simulink model "gm_wifi_server"  (R2015b)
settings: Solver=VariableStepAuto  StartTime=0.0  StopTime=10.0  RelTol=1e-3
settings Model: Creator=Administrator  LastModifiedBy=Administrator
settings OptimizationCC: BlockReduction=off  ConditionallyExecuteInputs=off
settings DebuggingCC: InheritedTsInSrcMsg=none

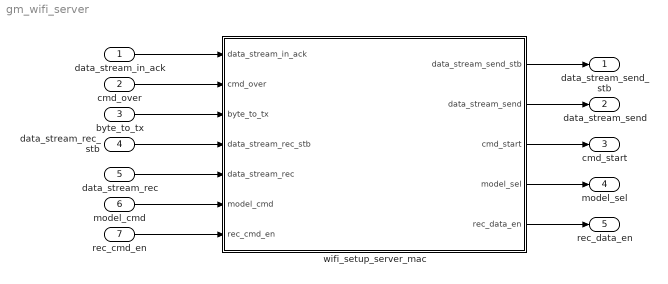
== system gm_wifi_server ==
  data_stream_in_ack : Inport  SampleTime=0
  cmd_over : Inport  Port=2  SampleTime=0
  byte_to_tx : Inport  Port=3  SampleTime=0
  data_stream_rec_stb : Inport  Port=4  SampleTime=0
  data_stream_rec : Inport  Port=5  SampleTime=0
  model_cmd : Inport  Port=6  SampleTime=0
  rec_cmd_en : Inport  Port=7  SampleTime=0
  wifi_setup_server_mac : Subsystem
  data_stream_send_stb : Outport
  data_stream_send : Outport  Port=2
  cmd_start : Outport  Port=3
  model_sel : Outport  Port=4
  rec_data_en : Outport  Port=5
  wires:
  data_stream_in_ack/1 -> wifi_setup_server_mac/1(data_stream_in_ack)
  cmd_over/1 -> wifi_setup_server_mac/2(cmd_over)
  byte_to_tx/1 -> wifi_setup_server_mac/3(byte_to_tx)
  data_stream_rec_stb/1 -> wifi_setup_server_mac/4(data_stream_rec_stb)
  data_stream_rec/1 -> wifi_setup_server_mac/5(data_stream_rec)
  model_cmd/1 -> wifi_setup_server_mac/6(model_cmd)
  rec_cmd_en/1 -> wifi_setup_server_mac/7(rec_cmd_en)
  wifi_setup_server_mac/1(data_stream_send_stb) -> data_stream_send_stb/1
  wifi_setup_server_mac/2(data_stream_send) -> data_stream_send/1
  wifi_setup_server_mac/3(cmd_start) -> cmd_start/1
  wifi_setup_server_mac/4(model_sel) -> model_sel/1
  wifi_setup_server_mac/5(rec_data_en) -> rec_data_en/1

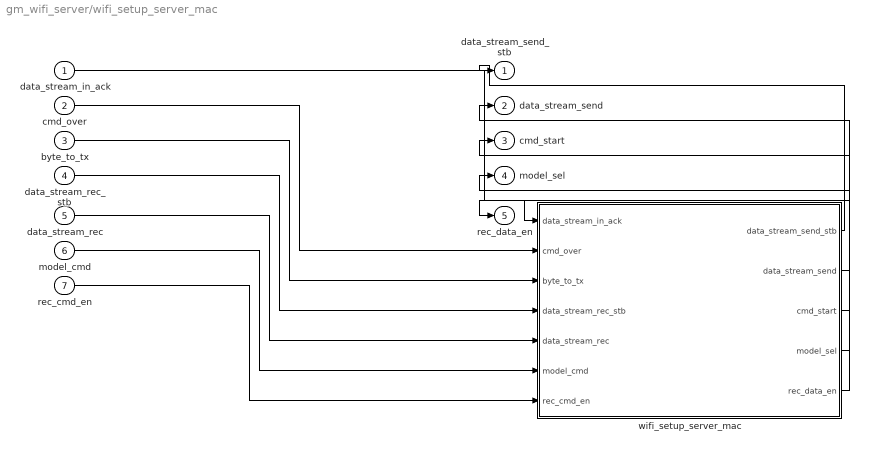
== system gm_wifi_server/wifi_setup_server_mac ==
  data_stream_in_ack : Inport  SampleTime=0
  cmd_over : Inport  Port=2  SampleTime=0
  byte_to_tx : Inport  Port=3  SampleTime=0
  data_stream_rec_stb : Inport  Port=4  SampleTime=0
  data_stream_rec : Inport  Port=5  SampleTime=0
  model_cmd : Inport  Port=6  SampleTime=0
  rec_cmd_en : Inport  Port=7  SampleTime=0
  wifi_setup_server_mac : Stateflow chart  TreatAsAtomicUnit=on
  data_stream_send_stb : Outport
  data_stream_send : Outport  Port=2
  cmd_start : Outport  Port=3
  model_sel : Outport  Port=4
  rec_data_en : Outport  Port=5
  wires:
  data_stream_in_ack/1 -> wifi_setup_server_mac/1(data_stream_in_ack)
  cmd_over/1 -> wifi_setup_server_mac/2(cmd_over)
  byte_to_tx/1 -> wifi_setup_server_mac/3(byte_to_tx)
  data_stream_rec_stb/1 -> wifi_setup_server_mac/4(data_stream_rec_stb)
  data_stream_rec/1 -> wifi_setup_server_mac/5(data_stream_rec)
  model_cmd/1 -> wifi_setup_server_mac/6(model_cmd)
  rec_cmd_en/1 -> wifi_setup_server_mac/7(rec_cmd_en)
  wifi_setup_server_mac/1(data_stream_send_stb) -> data_stream_send_stb/1
  wifi_setup_server_mac/2(data_stream_send) -> data_stream_send/1
  wifi_setup_server_mac/3(cmd_start) -> cmd_start/1
  wifi_setup_server_mac/4(model_sel) -> model_sel/1
  wifi_setup_server_mac/5(rec_data_en) -> rec_data_en/1

== stateflow chart gm_wifi_server/wifi_setup_server_mac/wifi_setup_server_mac ==
  settings: executeAtInitialization=1
  state initial
    entry:
    %outputs
    data_stream_send_stb=0;
    data_stream_send=0;
    cmd_start=0;
    model_sel=0;
    rec_data_en=0;
    %local variables
    cnt_wait=0;
    cnt_halt=0;
  state Tran1_A
    entry:
    data_stream_send_stb=1;
    data_stream_send=65;%A
    cnt_wait=0;
    cnt_halt=0;
  state Tran1_T
    entry:
    data_stream_send_stb=1;
    data_stream_send=84;%T
    cnt_wait=0;
    cnt_halt=0;
  state Tran1_Enter1
    entry:
    data_stream_send_stb=1;
    data_stream_send=10;%/n
    cnt_wait=0;
    cnt_halt=0;
  state Tran1_Enter
    entry:
    data_stream_send_stb=1;
    data_stream_send=13;%/r
    cnt_wait=0;
    cnt_halt=0;
  state send1_finish
    entry:
    data_stream_send_stb=0;
    data_stream_send=0;
    cnt_wait=0;
    cnt_halt=0;
  state wait1_cnt
    cnt_wait=cnt_wait+1;
    cnt_halt=0;
  state send_cmd1
    entry:
    %output
    cmd_start=1;
    data_stream_send_stb=0;
    data_stream_send=byte_to_tx;
    %local
    %cnt_wait=0;
    %cnt_halt=0;
  state send_cmd2
    entry:
    %output
    cmd_start=1;
    data_stream_send_stb=1;
    data_stream_send=byte_to_tx;
  state wait_cmd
    entry:
    cmd_start=1;
    data_stream_send_stb=1;
    data_stream_send=byte_to_tx;
  state device_OK
    entry:
    %output, start from 1
    model_sel=model_sel+1;
    cnt_wait=0;
  state send_cmd_over
    entry:
    cmd_start=0;
    data_stream_send_stb=0;
    data_stream_send=0;
  state Tran2_Enter
    entry:
    data_stream_send_stb=1;
    data_stream_send=13;%/r
  state Tran2_Enter1
    entry:
    data_stream_send_stb=1;
    data_stream_send=10;%/r
  state send2_finish
    entry:
    data_stream_send_stb=0;
    data_stream_send=0;
  state device_config_OK
    entry:
    model_sel=6;
    cnt_halt=0;
  state wait_port
    entry:
    rec_data_en=0;
    cnt_halt=cnt_halt+1;
  state wait_server_rec_S
    entry:
    cnt_halt=cnt_halt+1;
  state wait_server_rec_T
    entry:
    rec_data_en=1;
    %when get T, begin rec data
  state rec_data
    entry:
    cnt_halt=cnt_halt+1;
  state pre_rec_data
  state send_word
    entry:
    cmd_start=1;
    data_stream_send_stb=0;
    data_stream_send=byte_to_tx;
    cnt_halt=0;
  state send_word1
    entry:
    cmd_start=1;
    data_stream_send_stb=1;
    data_stream_send=byte_to_tx;
  state wait_data
    entry:
    cmd_start=1;
    data_stream_send_stb=1;
    data_stream_send=byte_to_tx;
  state begin_send_data
    entry:
    model_sel=7;
    cnt_halt=0;
  state send_data_over
    entry:
    cmd_start=0;
    data_stream_send_stb=0;
    data_stream_send=0;
  state Tran3_Enter
    entry:
    data_stream_send_stb=1;
    data_stream_send=13;%/r
  state Tran3_Enter1
    entry:
    data_stream_send_stb=1;
    data_stream_send=10;%/r
  state send3_finish
    entry:
    data_stream_send_stb=0;
    data_stream_send=0;
  state data_send_over
    entry:
    model_sel=7;
    cnt_halt=0;
  (default) -> initial
  initial -> Tran1_A
  Tran1_A -> (junction 17)
  (junction 17) -> Tran1_T [order 2] : [data_stream_in_ack==1]
  Tran1_T -> (junction 29)
  (junction 29) -> Tran1_Enter [order 1] : [data_stream_in_ack==1]
  Tran1_Enter -> (junction 31)
  (junction 31) -> Tran1_Enter1 [order 1] : [data_stream_in_ack==1]
  (junction 29) -> Tran1_T [order 2] : [data_stream_in_ack==0]
  (junction 31) -> Tran1_Enter [order 2] : [data_stream_in_ack==0]
  (junction 17) -> Tran1_A [order 1] : [data_stream_in_ack==0]
  (junction 42) -> Tran1_Enter1 [order 1] : [data_stream_in_ack==0]
  (junction 49) -> Tran1_A [order 1] : [model_cmd~=1]
  Tran1_Enter1 -> (junction 42)
  (junction 42) -> send1_finish [order 2] : [data_stream_in_ack==1]
  (junction 46) -> (junction 49) [order 2] : [rec_cmd_en==1]
  send1_finish -> (junction 46)
  (junction 46) -> send1_finish [order 1] : [rec_cmd_en==0]
  (junction 49) -> wait1_cnt [order 2] : [model_cmd==1]
  (junction 54) -> wait1_cnt [order 1] : [cnt_wait<5000000]
      | %0.5s
  wait1_cnt -> (junction 54)
  (junction 97) -> wait1_cnt
  (junction 63) -> send_cmd2 [order 1] : [data_stream_in_ack==0]
  (junction 81) -> Tran2_Enter [order 1] : [data_stream_in_ack==0]
  (junction 54) -> (junction 100) [order 2] : [cnt_wait>=5000000]%0.5s
  (junction 85) -> Tran2_Enter1 [order 1] : [data_stream_in_ack==0]
  send_cmd2 -> (junction 63)
  (junction 63) -> wait_cmd [order 2] : [data_stream_in_ack==1]
  wait_cmd -> (junction 70)
  (junction 70) -> send_cmd_over [order 2] : [cmd_over==1]
  send_cmd_over -> Tran2_Enter
  Tran2_Enter -> (junction 81)
  (junction 81) -> Tran2_Enter1 [order 2] : [data_stream_in_ack==1]
  send_cmd1 -> send_cmd2
  device_OK -> send_cmd1
  (junction 70) -> (junction 76) [order 1] : [cmd_over==0]
  (junction 100) -> device_OK [order 1] : [model_sel~=5]
  (junction 100) -> device_config_OK [order 2] : [model_sel==5]
  (junction 76) -> send_cmd1
  Tran2_Enter1 -> (junction 85)
  (junction 94) -> send_cmd1 [order 1] : [model_cmd~=1]
      | %This command does not config sucessfully.
  (junction 85) -> send2_finish [order 2] : [data_stream_in_ack==1]
  send2_finish -> (junction 91)
  (junction 91) -> (junction 94) [order 2] : [rec_cmd_en==1]
  (junction 91) -> send2_finish [order 1] : [rec_cmd_en==0]
  (junction 94) -> (junction 97) [order 2] : [model_cmd==1]
  (junction 120) -> pre_rec_data [order 2] : [data_stream_rec_stb==0]
  device_config_OK -> (junction 104)
  (junction 104) -> wait_server_rec_S [order 1] : [(data_stream_rec_stb==1)&&(data_stream_rec==83)]
      | %when receive S from client
  wait_server_rec_S -> (junction 109)
  (junction 109) -> wait_server_rec_T [order 1] : [(data_stream_rec_stb==1)&&(data_stream_rec==84)]
      | %when receive T from client
  (junction 129) -> wait_port [order 1] : [cnt_halt<=2000000]%0.02s
  (junction 104) -> device_config_OK [order 2] : [(data_stream_rec_stb~=1)||(data_stream_rec~=83)]
  pre_rec_data -> (junction 120)
  (junction 120) -> rec_data [order 1] : [data_stream_rec_stb==1]
  rec_data -> (junction 124)
  (junction 124) -> wait_port [order 2] : [cnt_halt==8]
      | {cnt_halt=0;}
  wait_server_rec_T -> pre_rec_data : {cnt_halt=0;}
  (junction 109) -> (junction 113) [order 2] : [(data_stream_rec_stb~=1)||(data_stream_rec~=84)]
  (junction 124) -> pre_rec_data [order 1] : [cnt_halt<8]
  (junction 113) -> wait_server_rec_S [order 1] : [cnt_halt<=500000000]%5sec
  (junction 172) -> device_config_OK
  (junction 113) -> device_config_OK [order 2] : [cnt_halt>500000000]%5sec
  wait_port -> (junction 129)
  (junction 129) -> send_word [order 2] : [cnt_halt>2000000]%0.02s
  (junction 136) -> send_word1 [order 2] : [data_stream_in_ack==0]
  send_word -> send_word1
  (junction 136) -> wait_data [order 1] : [data_stream_in_ack==1]
  send_word1 -> (junction 136)
  wait_data -> (junction 141)
  (junction 141) -> send_word [order 1] : [cmd_over==0]
  (junction 166) -> send_word [order 1] : [model_cmd~=1]
  begin_send_data -> send_word
  (junction 141) -> send_data_over [order 2] : [cmd_over==1]
  (junction 155) -> Tran3_Enter [order 1] : [data_stream_in_ack==0]
  (junction 155) -> Tran3_Enter1 [order 2] : [data_stream_in_ack==1]
  Tran3_Enter -> (junction 155)
  send_data_over -> Tran3_Enter
  (junction 166) -> begin_send_data [order 2] : [model_cmd==1]
  (junction 148) -> Tran3_Enter1 [order 1] : [data_stream_in_ack==0]
  Tran3_Enter1 -> (junction 148)
  (junction 161) -> send3_finish [order 1] : [rec_cmd_en==0]
  (junction 148) -> send3_finish [order 2] : [data_stream_in_ack==1]
  send3_finish -> (junction 159)
  (junction 159) -> (junction 161) [order 1] : [model_sel~=7]
  (junction 161) -> (junction 166) [order 2] : [rec_cmd_en==1]
  (junction 159) -> data_send_over [order 2] : [model_sel==7]
  data_send_over -> (junction 172)
  data: data_stream_in_ack input boolean; cmd_over input boolean; byte_to_tx input uint8; data_stream_rec_stb input boolean; data_stream_rec input uint8; model_cmd input fixdt(0,4,0); rec_cmd_en input boolean; data_stream_send_stb output boolean; data_stream_send output uint8; cmd_start output boolean; model_sel output fixdt(0,4,0); rec_data_en output boolean; cnt_wait local uint32; cnt_halt local int32
